simulink model "rev_eee_train"  (R2024a)
settings: Solver=VariableStepAuto  StartTime=0.0  StopTime=2  RelTol=1e-3
libraries: spsSeriesRLCBranchLib x9, spsVoltageMeasurementLib x6, spsBreakerLib x3, spsDiodeLib x1, spsIGBTDiodeLib x1, spsPLLLib x1, spsPVArrayLib x1, spsPWMGenerator2LevelLib x1, spsPWMGeneratorDCDCLib x1, rllib x1, spsUniversalBridgeLib x1, sps_lib x1
settings Model: Creator=megha  LastModifiedBy=megha

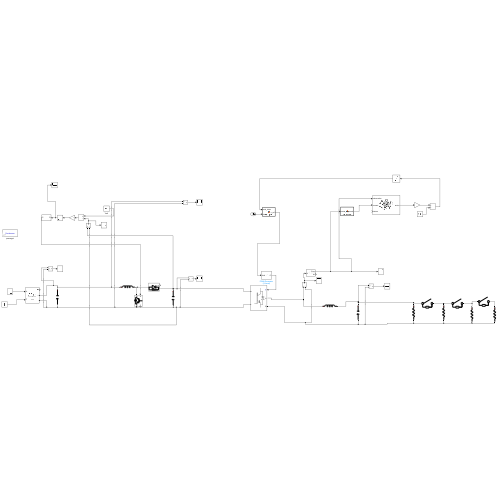
[thumbnail: Simulink's stored preview of the top-level diagram]
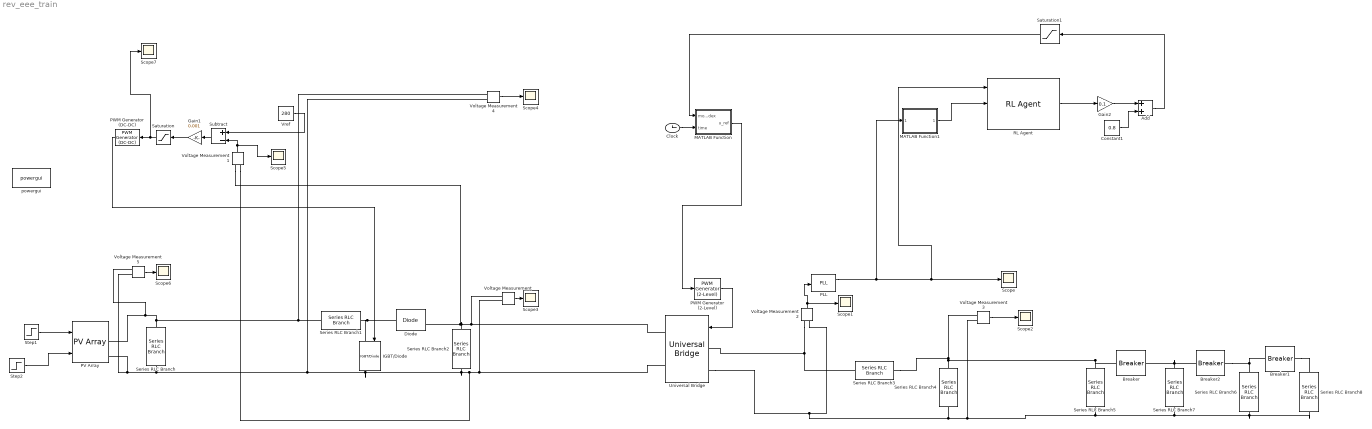
== system rev_eee_train ==
  Add : Sum
  Breaker : spsBreakerLib/Breaker  InitialState=0  SwitchingTimes="[9  18]"  External=off  BreakerResistance=0.01  SnubberResistance=1e6  SnubberCapacitance=inf  Measurements=None  MoreParameters=on  NoBreakLoop=off
  Breaker1 : spsBreakerLib/Breaker  InitialState=0  SwitchingTimes=[4 10]  External=off  BreakerResistance=0.01  SnubberResistance=1e6  SnubberCapacitance=inf  Measurements=None  MoreParameters=on  NoBreakLoop=off
  Breaker2 : spsBreakerLib/Breaker  InitialState=0  SwitchingTimes=[2 14]  External=off  BreakerResistance=0.01  SnubberResistance=1e6  SnubberCapacitance=inf  Measurements=None  MoreParameters=on  NoBreakLoop=off
  Clock : Clock
  Constant1 : Constant  Value=0.8
  Diode : spsDiodeLib/Diode  Ron=0.001  Lon=0  Vf=0.8  IC=0  UseSnubber=0  Rs=500  Cs=250e-9  Measurements=on
  Gain1 : Gain  Gain=0.001
  Gain2 : Gain  Gain=0.1
  IGBT/Diode : spsIGBTDiodeLib/IGBT//Diode  Ron=1e-3  Rs=1e5  Cs=inf  Measurements=on
  MATLAB Function : MATLAB Function  TreatAsAtomicUnit=on
  MATLAB Function1 : MATLAB Function  TreatAsAtomicUnit=on
  PLL : spsPLLLib/PLL  Fmin=45  Par_Init=[0, 60]  ParK=[180, 500, 1]  TcD=1e-4  MaxRateChangeFreq=60  FilterCutOffFreq=15  Ts=0  AGC=on
      settings: LibrarySourceBlock=sps_lib/Control/PLL
  PV Array : spsPVArrayLib/PV Array  Npar=40  Nser=4  PlotType=array @ 1000 W/m2 & specified temperatures  S_vec="[ 1000  500  100 ]"  Temp_C_vec="[ 45 25  ]"  ModuleName=User-defined  PlotWhenSelected=off  Pm=213.15  Ncell=60  Voc=36.3  Isc=7.84  Vm=29  Im=7.35  beta_Voc_pc=-0.36099  alpha_Isc_pc=0.102  beta_Voc=-0.13104  alpha_Isc=0.0079968  IL=7.8654  I0=2.9273e-10  nI=0.98119  Rsh=313.0553  Rs=0.39381  RobustModel=off  RobustCellTemperature=313.3991  BAL=on  Tc=1e-6  Tfilter=5e-5
  PWM Generator (2-Level) : spsPWMGenerator2LevelLib/PWM Generator (2-Level)  ModulatorType=Single-phase full-bridge (4 pulses)  ModulatorMode=Unsynchronized  Fc=27*60  Pc=90  nF=27  MinMax="[ -1  1 ]"  SamplingTechnique=Natural  ModulatingSignals=off  m=0.8  Freq=60  Phase=0  Ts=0  ShowCarrierOutport=off
  PWM Generator (DC-DC) : spsPWMGeneratorDCDCLib/PWM Generator (DC-DC)  Fsw=1500  Ts=0
  RL Agent : rllib/RL Agent  Agent=agent  ExternalActionAsInput=off  ProvideLastAction=off  ProvideCumRwd=off  TreatAsDirectFeedthrough=on  UseStrictObservationDataTypes=off
  Saturation : Saturate  UpperLimit=1  LowerLimit=0
  Saturation1 : Saturate  UpperLimit=1  LowerLimit=0.65
  Scope{,1..7} (8 alike) : Scope
  Series RLC Branch : spsSeriesRLCBranchLib/Series RLC Branch  LConnTagsString=__new0  RConnTagsString=__new0  BranchType=C  Resistance=1  Inductance=1e-3  SetiL0=off  InitialCurrent=0  Capacitance=0.006  Setx0=off  InitialVoltage=0  Measurements=None
  Series RLC Branch1 : spsSeriesRLCBranchLib/Series RLC Branch  LConnTagsString=__new0  RConnTagsString=__new0  BranchType=L  Resistance=1  Inductance=0.02  SetiL0=off  InitialCurrent=0  Capacitance=1e-6  Setx0=off  InitialVoltage=0  Measurements=None
  Series RLC Branch2 : spsSeriesRLCBranchLib/Series RLC Branch  LConnTagsString=__new0  RConnTagsString=__new0  BranchType=C  Resistance=1  Inductance=1e-3  SetiL0=off  InitialCurrent=0  Capacitance=0.006  Setx0=off  InitialVoltage=0  Measurements=None
  Series RLC Branch3 : spsSeriesRLCBranchLib/Series RLC Branch  LConnTagsString=__new0  RConnTagsString=__new0  BranchType=L  Resistance=1  Inductance=0.02  SetiL0=off  InitialCurrent=0  Capacitance=1e-6  Setx0=off  InitialVoltage=0  Measurements=None
  Series RLC Branch4 : spsSeriesRLCBranchLib/Series RLC Branch  LConnTagsString=__new0  RConnTagsString=__new0  BranchType=C  Resistance=1  Inductance=1e-3  SetiL0=off  InitialCurrent=0  Capacitance=0.006  Setx0=off  InitialVoltage=0  Measurements=None
  Series RLC Branch5 : spsSeriesRLCBranchLib/Series RLC Branch  LConnTagsString=__new0  RConnTagsString=__new0  BranchType=R  Resistance=100  Inductance=1e-3  SetiL0=off  InitialCurrent=0  Capacitance=1e-6  Setx0=off  InitialVoltage=0  Measurements=None
  Series RLC Branch6 : spsSeriesRLCBranchLib/Series RLC Branch  LConnTagsString=__new0  RConnTagsString=__new0  BranchType=R  Resistance=10  Inductance=1e-3  SetiL0=off  InitialCurrent=0  Capacitance=1e-6  Setx0=off  InitialVoltage=0  Measurements=None
  Series RLC Branch7 : spsSeriesRLCBranchLib/Series RLC Branch  LConnTagsString=__new0  RConnTagsString=__new0  BranchType=R  Resistance=30  Inductance=0.005  SetiL0=off  InitialCurrent=0  Capacitance=1e-6  Setx0=off  InitialVoltage=0  Measurements=None
  Series RLC Branch8 : spsSeriesRLCBranchLib/Series RLC Branch  LConnTagsString=__new0  RConnTagsString=__new0  BranchType=R  Resistance=110  Inductance=1e-3  SetiL0=off  InitialCurrent=0  Capacitance=1e-6  Setx0=off  InitialVoltage=0  Measurements=None
  Step1 : Step  Time=0.5  Before=1000  After=800  SampleTime=0
  Step2 : Step  Before=25  After=32  SampleTime=0
  Subtract : Sum  Inputs=+-
  Universal Bridge : spsUniversalBridgeLib/Universal Bridge  Arms=2  SnubberResistance=1e5  SnubberCapacitance=inf  Device=IGBT / Diodes  Ron=1e-3  Lon=0  ForwardVoltages="[  0  0  ]"  ForwardVoltage=0  GTOparameters=[ 10e-6 , 20e-6 ]  IGBTparameters=[ 1e-6 , 2e-6 ]  Measurements=None  Measurements_2=None  converterType=Rectifier
  Voltage Measurement{,1..5} (6 alike) : spsVoltageMeasurementLib/Voltage Measurement  PhasorSimulation=off  OutputType=Complex  PSBequivalent=0
  Vref : Constant  Value=280
  powergui : sps_lib/powergui  Priority=1  SimulationMode=Continuous  SampleTime=50e-6  frequency=60  Iterations=50  frequencyindice=0  Pbase=100e6  ErrMax=1e-4  UnitsV=kV  UnitsW=MW  buscounter=0  FunctionMessages=off  echomessages=off  EnableUseOfTLC=off  CurrentSourceSwitches=off  DisableSnubberDevices=off  DisableRonSwitches=off  DisableVfSwitches=off  DisplayEquations=off  AutomaticDiscreteSolvers=off  SolverType=Tustin/Backward Euler (TBE)  Interpol=off  ExternalGateDelay=off  methode=off  Ts=100  x0status=blocks  SPID=on  SwTol=0  HookPort=off  NonlinearTolerance=1e-4  nMaxIteration=100  ContinueOnMaxIteration=off  RestoreLinks=warning  ResistiveCurrentMeasurement=off  Frange=[0:2:500]  Ylog=off  Xlog=on  ShowGrid=off  save=off  variable=ZData  structure=0  ZoomFFT=off  StartTime=0.0  cycles=1  DisplayStyle=1  fundamental=60  FreqAxis=off  MaxFrequency=1000  frequencyindicesteady=1  RmsSteady=1  display=off
  wires:
  Voltage Measurement/1 -> Scope3/1
  PWM Generator (2-Level)/1 -> Universal Bridge/1
  Voltage Measurement1/1 -> Scope5/1, Subtract/2
  Voltage Measurement2/1 -> Scope1/1, PLL/1
  Subtract/1 -> Gain1/1
  Voltage Measurement3/1 -> Scope2/1
  PWM Generator (DC-DC)/1 -> IGBT/Diode/1
  Gain1/1 -> Saturation/1
  Vref/1 -> Subtract/1
  Saturation/1 -> Scope7/1, PWM Generator (DC-DC)/1
  PLL/1 -> RL Agent/1, Scope/1, MATLAB Function1/1(meas_freq)
  MATLAB Function1/1(reward) -> RL Agent/2
  RL Agent/1 -> Gain2/1
  Gain2/1 -> Add/1
  Constant1/1 -> Add/2
  Add/1 -> Saturation1/1
  MATLAB Function/1(u_ref) -> PWM Generator (2-Level)/1
  Saturation1/1 -> MATLAB Function/1(mod_index)
  Clock/1 -> MATLAB Function/2(time)
  Voltage Measurement4/1 -> Scope4/1
  Voltage Measurement5/1 -> Scope6/1
  Step1/1 -> PV Array/1
  Step2/1 -> PV Array/2
  connections:
  Series RLC Branch3/RConn1 -- Voltage Measurement3/LConn1 -- Breaker/LConn1 -- Series RLC Branch5/LConn1 -- Series RLC Branch4/LConn1
  Diode/RConn1 -- Series RLC Branch2/LConn1 -- Voltage Measurement/LConn1 -- Universal Bridge/RConn1 -- Voltage Measurement1/LConn1
  Series RLC Branch1/RConn1 -- Diode/LConn1 -- IGBT/Diode/LConn1
  Voltage Measurement1/LConn2 -- Voltage Measurement/LConn2 -- Universal Bridge/RConn2 -- Voltage Measurement4/LConn2 -- Series RLC Branch/RConn1 -- Voltage Measurement5/LConn2 -- PV Array/RConn2 -- IGBT/Diode/RConn1 -- Series RLC Branch2/RConn1
  Series RLC Branch1/LConn1 -- Series RLC Branch/LConn1 -- Voltage Measurement5/LConn1 -- PV Array/RConn1 -- Voltage Measurement4/LConn1
  Series RLC Branch4/RConn1 -- Universal Bridge/LConn2 -- Voltage Measurement2/LConn2 -- Voltage Measurement3/LConn2 -- Series RLC Branch5/RConn1 -- Series RLC Branch8/RConn1 -- Series RLC Branch6/RConn1 -- Series RLC Branch7/RConn1
  Breaker2/LConn1 -- Series RLC Branch7/LConn1 -- Breaker/RConn1
  Universal Bridge/LConn1 -- Series RLC Branch3/LConn1 -- Voltage Measurement2/LConn1
  Breaker2/RConn1 -- Breaker1/LConn1 -- Series RLC Branch6/LConn1
  Breaker1/RConn1 -- Series RLC Branch8/LConn1

== matlab function rev_eee_train/MATLAB Function ==
  data: mod_index input; u_ref output; time input
function u_ref = ref_gen(mod_index, time)
    % Generates a 60 Hz sine wave scaled by modulation index
    freq = 60; % Hz
    u_ref = mod_index * sin(2 * pi * freq * time);
end

== matlab function rev_eee_train/MATLAB Function1 ==
  data: meas_freq input; reward output
function reward = calc_reward(meas_freq)
    % Ensure freq_dev is properly defined
    freq_dev = meas_freq - 60;  % Calculate the frequency deviation from 60 Hz

    % Penalize frequency deviation (squared for smooth optimization)
    freq_penalty = -freq_dev^2;  

    % Stability bonus (closer to zero deviation is better)
    stability_reward = 1 - abs(freq_dev);  % Max reward = 1, min < 0

    % Combined reward function
    reward = freq_penalty + stability_reward;
end
